simulink model "GNC"  (R2015a)
settings: Solver=ode45  StartTime=0.0  StopTime=10.0  RelTol=1e-3
settings Model: Creator=Andrew  LastModifiedBy=Andrew

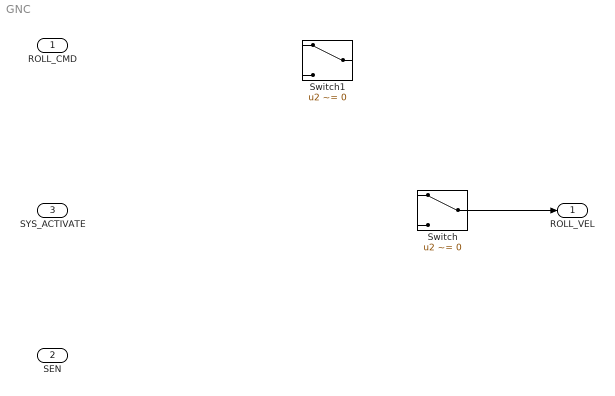
== system GNC ==
  ROLL_CMD : Inport
  SEN : Inport  Port=2
  SYS_ACTIVATE : Inport  Port=3
  Switch : Switch  Criteria=u2 ~= 0
  Switch1 : Switch  Criteria=u2 ~= 0
  ROLL_VEL : Outport
  wires:
  Switch/1 -> ROLL_VEL/1
